simulink model "MECN4029_SIMULINK_BLOCKS_DIAGRAMS"  (R2023b)
settings: Solver=VariableStepAuto  StartTime=0.0  StopTime=815  RelTol=1e-3
PreLoadFcn:
  | Kg=2000;
  | Kt=0.05;
  | Kf=0.05;
  | L=0.006;
  | R=3;
  | J=2.3491;
  | l=1.722;
  | w=1.134;
  | t=0.035;
  | m=21.9;
  | Kd=5;
libraries: slpidlib x2, simulink x1
settings Model: Creator=user  LastModifiedBy=user
settings DataIOCC: ExternalInput=[summertime summerposition]  LoadExternalInput=on

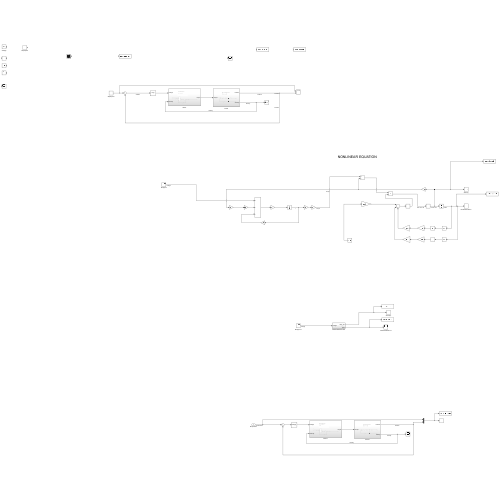
[thumbnail: Simulink's stored preview of the top-level diagram]
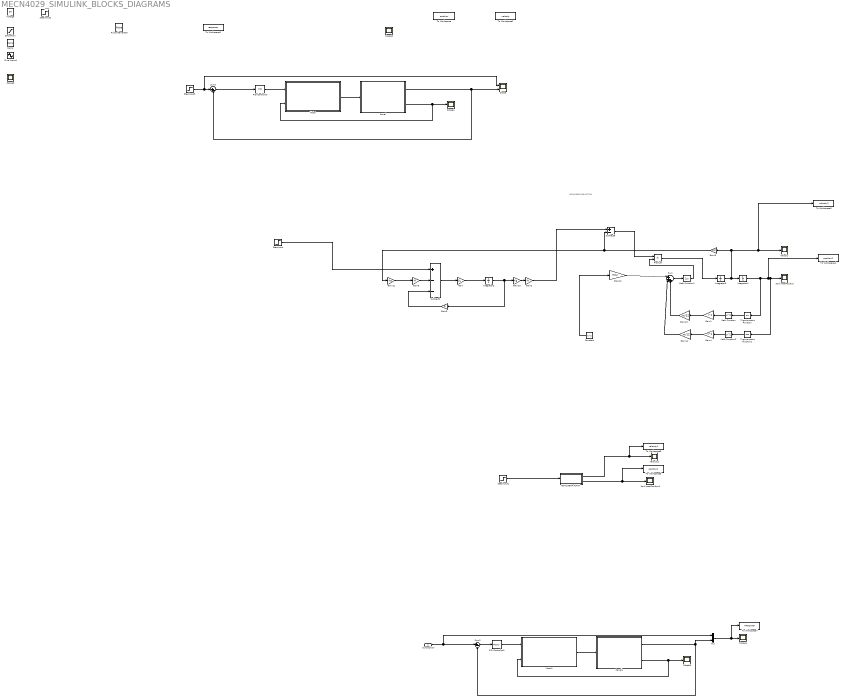
== system MECN4029_SIMULINK_BLOCKS_DIAGRAMS ==
  note: NONLINEAR EQUATION
  Sunposition : Inport
  Constant : Constant  Value=w^2
  Gain : Gain  Gain=1/L
  Gain1 : Gain  Gain=l^2
  Gain10 : Gain  Gain=Kg
  Gain11 : Gain  Gain=Kg
  Gain12 : Gain  Gain=m/12
  Gain13 : Gain  Gain=m/12
  Gain14 : Gain  Gain=m/12
  Gain2 : Gain  Gain=Kt
  Gain3 : Gain  Gain=R
  Gain4 : Gain  Gain=t^2
  Gain5 : Gain  Gain=Kf
  Gain8 : Gain  Gain=Kd
  Integrator1 : Integrator
  Integrator2 : Integrator
  Integrator3 : Integrator
  Math Function : Math  Operator=square
  Math Function1 : Math  Operator=reciprocal
  Math Function2 : Math  Operator=square
  Motor : Subsystem
  Motor1 : Subsystem
  Mux : Mux  Inputs=2
  NON-LINEAR PLANT : Subsystem
  NonlinearPosition : Scope
  NonlinearPosition1 : Scope
  PID Controller : slpidlib/PID Controller  Controller=P  Form=Parallel  TimeDomain=Continuous-time  UseExternalTs=off  SampleTime=-1  IntegratorMethod=Forward Euler  FilterMethod=Forward Euler  ControllerParametersSource=internal  P=200  I=1  UseKiTs=off  D=0  N=100  UseFilter=on  TunerSelectOption=Transfer Function Based (PID Tuner App)  InitialConditionSource=internal  InitialConditionForIntegrator=0  InitialConditionForFilter=0  DifferentiatorICPrevScaledInput=0  ExternalReset=none  TrackingMode=off  Kt=1  LimitOutput=off  SatLimitsSource=internal  UpperSaturationLimit=inf  LowerSaturationLimit=-inf  LinearizeAsGain=on  AntiWindupMode=none  Kb=1  LimitIntegrator=off  UpperIntegratorSaturationLimit=inf  LowerIntegratorSaturationLimit=-inf  POutMin=[]  POutMax=[]  IOutMin=[]  IOutMax=[]  DOutMin=[]  DOutMax=[]  NOutMin=[]  NOutMax=[]  SumOutMin=[]  SumOutMax=[]  SaturationOutMin=[]  SaturationOutMax=[]  PParamMin=[]  PParamMax=[]  IParamMin=[]  IParamMax=[]  DParamMin=[]  DParamMax=[]  NParamMin=[]  NParamMax=[]  KbParamMin=[]  KbParamMax=[]  KtParamMin=[]  KtParamMax=[]  KbOutMin=[]  KbOutMax=[]  KtOutMin=[]  KtOutMax=[]  IntegratorOutMin=[]  IntegratorOutMax=[]  FilterOutMin=[]  FilterOutMax=[]  SumI1OutMin=[]  SumI1OutMax=[]  SumI2OutMin=[]  SumI2OutMax=[]  SumI3OutMin=[]  SumI3OutMax=[]  SumI4OutMin=[]  SumI4OutMax=[]  SumDOutMin=[]  SumDOutMax=[]  DifferentiatorOutMin=[]  DifferentiatorOutMax=[]  FilterDiffOutCoefMin=[]  FilterDiffOutCoefMax=[]  ReciprocalOutMin=[]  ReciprocalOutMax=[]  SumDenOutMin=[]  SumDenOutMax=[]  SumNumOutMin=[]  SumNumOutMax=[]  DivideOutMin=[]  DivideOutMax=[]  UdiffTsProdOutMin=[]  UdiffTsProdOutMax=[]  NTsProdOutMin=[]  NTsProdOutMax=[]  UintegralTsProdOutMin=[]  UintegralTsProdOutMax=[]  UngainTsProdOutMin=[]  UngainTsProdOutMax=[]  ClampingZeroOutDataTypeStr=Inherit: Inherit via back propagation  ClampingZeroOutMin=[]  ClampingZeroOutMax=[]  FilterDenConstantOutDataTypeStr=Inherit: Inherit via back propagation  FilterDenConstantOutMin=[]  FilterDenConstantOutMax=[]  PCopyOutDataTypeStr=Inherit: Inherit via back propagation  PCopyOutMin=[]  PCopyOutMax=[]  NCopyOutDataTypeStr=Inherit: Inherit via back propagation  NCopyOutMin=[]  NCopyOutMax=[]  IntegratorContinuousStateAttributes=''  IntegratorStateMustResolveToSignalObject=off  IntegratorRTWStateStorageClass=Auto  FilterContinuousStateAttributes=''  FilterStateMustResolveToSignalObject=off  FilterRTWStateStorageClass=Auto  ParallelPVariant=InternalParameters  IdealPVariant=Disabled  IVariant=Disabled  DVariant=Disabled  IntegratorVariant=Disabled  SatVariant=Disabled  AWVariant=Disabled  PCopyVariant=Disabled  TRVariant=Disabled  FdbkBlocksVariant=Forward  IdealPFdbkVariant=Disabled  SatFdbkVariant=Disabled  DerivativeFilterVariant=Disabled  NVariant=Disabled  NCopyVariant=Disabled_SignalSpec  FilterICVariant=Disabled  IntegratorICVariant=Disabled  ExternalResetVariant=Disabled  TRSumVariant=Passthrough  SumFdbkVariant=Disabled  SumVariant=Passthrough_P  TsampFilterVariant=InternalTs  TsampNgainVariant=Passthrough  TsampIntegralVariant=Disabled_SignalSpec  ExternalSaturationOutDataTypeStr=Inherit: Same as second input
  PID Controller1 : slpidlib/PID Controller  Controller=PID  Form=Parallel  TimeDomain=Continuous-time  UseExternalTs=off  SampleTime=-1  IntegratorMethod=Forward Euler  FilterMethod=Forward Euler  ControllerParametersSource=internal  P=4922.7881  I=45069.5184  UseKiTs=off  D=-17.6742  N=85.9588  UseFilter=on  TunerSelectOption=Transfer Function Based (PID Tuner App)  InitialConditionSource=internal  InitialConditionForIntegrator=0  InitialConditionForFilter=0  DifferentiatorICPrevScaledInput=0  ExternalReset=none  TrackingMode=off  Kt=1  LimitOutput=off  SatLimitsSource=internal  UpperSaturationLimit=inf  LowerSaturationLimit=-inf  LinearizeAsGain=on  AntiWindupMode=none  Kb=1  LimitIntegrator=off  UpperIntegratorSaturationLimit=inf  LowerIntegratorSaturationLimit=-inf  POutMin=[]  POutMax=[]  IOutMin=[]  IOutMax=[]  DOutMin=[]  DOutMax=[]  NOutMin=[]  NOutMax=[]  SumOutMin=[]  SumOutMax=[]  SaturationOutMin=[]  SaturationOutMax=[]  PParamMin=[]  PParamMax=[]  IParamMin=[]  IParamMax=[]  DParamMin=[]  DParamMax=[]  NParamMin=[]  NParamMax=[]  KbParamMin=[]  KbParamMax=[]  KtParamMin=[]  KtParamMax=[]  KbOutMin=[]  KbOutMax=[]  KtOutMin=[]  KtOutMax=[]  IntegratorOutMin=[]  IntegratorOutMax=[]  FilterOutMin=[]  FilterOutMax=[]  SumI1OutMin=[]  SumI1OutMax=[]  SumI2OutMin=[]  SumI2OutMax=[]  SumI3OutMin=[]  SumI3OutMax=[]  SumI4OutMin=[]  SumI4OutMax=[]  SumDOutMin=[]  SumDOutMax=[]  DifferentiatorOutMin=[]  DifferentiatorOutMax=[]  FilterDiffOutCoefMin=[]  FilterDiffOutCoefMax=[]  ReciprocalOutMin=[]  ReciprocalOutMax=[]  SumDenOutMin=[]  SumDenOutMax=[]  SumNumOutMin=[]  SumNumOutMax=[]  DivideOutMin=[]  DivideOutMax=[]  UdiffTsProdOutMin=[]  UdiffTsProdOutMax=[]  NTsProdOutMin=[]  NTsProdOutMax=[]  UintegralTsProdOutMin=[]  UintegralTsProdOutMax=[]  UngainTsProdOutMin=[]  UngainTsProdOutMax=[]  ClampingZeroOutDataTypeStr=Inherit: Inherit via back propagation  ClampingZeroOutMin=[]  ClampingZeroOutMax=[]  FilterDenConstantOutDataTypeStr=Inherit: Inherit via back propagation  FilterDenConstantOutMin=[]  FilterDenConstantOutMax=[]  PCopyOutDataTypeStr=Inherit: Inherit via back propagation  PCopyOutMin=[]  PCopyOutMax=[]  NCopyOutDataTypeStr=Inherit: Inherit via back propagation  NCopyOutMin=[]  NCopyOutMax=[]  IntegratorContinuousStateAttributes=''  IntegratorStateMustResolveToSignalObject=off  IntegratorRTWStateStorageClass=Auto  FilterContinuousStateAttributes=''  FilterStateMustResolveToSignalObject=off  FilterRTWStateStorageClass=Auto  ParallelPVariant=InternalParameters  IdealPVariant=Disabled  IVariant=InternalParameters  DVariant=InternalParameters  IntegratorVariant=Continuous  SatVariant=Disabled  AWVariant=Passthrough  PCopyVariant=Disabled  TRVariant=Disabled  FdbkBlocksVariant=Forward  IdealPFdbkVariant=Disabled  SatFdbkVariant=Disabled  DerivativeFilterVariant=ContFilter  NVariant=InternalParameters  NCopyVariant=Disabled  FilterICVariant=InternalICsFilter  IntegratorICVariant=InternalICs  ExternalResetVariant=Disabled  TRSumVariant=Passthrough  SumFdbkVariant=Disabled  SumVariant=Sum_PID  TsampFilterVariant=InternalTs  TsampNgainVariant=Passthrough  TsampIntegralVariant=Disabled_SignalSpec  ExternalSaturationOutDataTypeStr=Inherit: Same as second input
  Panel : Subsystem
  Panel1 : Subsystem
  Product : Product
  Pulse Generator : DiscretePulseGenerator  PulseType=Time based  Amplitude=30  Period=0.05  PulseWidth=5  PhaseDelay=0.01  VectorParams1D=off
  Ramp : simulink/Sources/Ramp  slope=5  start=1  InitialOutput=0
  Saturation : Saturate  UpperLimit=30  LowerLimit=-30
  Scope : Scope  NumInputPorts=2
  Scope{1..5} (5 alike) : Scope
  Sine Wave1 : Sin  Amplitude=30  SampleTime=0
  StepInput : Step  Time=0.01  After=30  SampleTime=0
  StepInput1 : Step  Time=0.01  After=30  SampleTime=0
  StepInput2 : Step  Time=0.01  After=30  SampleTime=0
  StepInput3 : Step  After=30  SampleTime=0
  Subtract1 : Sum  Inputs=+--
  Subtract3 : Sum  Inputs=+-
  Sum : Sum  Inputs=|+++  OutDataTypeStr=Inherit: Keep MSB
  Sum1 : Sum  Inputs=|+-
  Sum2 : Sum  Inputs=|+-
  To Workspace : ToWorkspace  VariableName=position  SampleTime=-1
  To Workspace1 : ToWorkspace  VariableName=velocity  SampleTime=-1
  To Workspace2 : ToWorkspace  VariableName=response  SampleTime=-1
  To Workspace3 : ToWorkspace  VariableName=velocity2  SampleTime=-1
  To Workspace4 : ToWorkspace  VariableName=position2  SampleTime=-1
  To Workspace5 : ToWorkspace  VariableName=velocity1  SampleTime=-1
  To Workspace6 : ToWorkspace  VariableName=position1  SampleTime=-1
  To Workspace7 : ToWorkspace  VariableName=TRACKING  SampleTime=-1
  Trigonometric Function : Trigonometry
  Trigonometric Function1 : Trigonometry  Operator=cos
  Velocity : Scope
  Velocity1 : Scope
  Voltage : Constant  Value=30
  wires:
  Panel/1(Position) -> Sum1/2, Scope/2  "Position"
  Panel/2(Velocity) -> Scope1/1, Motor/2(Velocity)  "Velocity"
  Motor/1(torque) -> Panel/1(Torque)
  Integrator1/1 -> Trigonometric Function/1, To Workspace4/1, Trigonometric Function1/1, NonlinearPosition/1  "theta"
  Integrator3/1 -> Gain8/1, To Workspace3/1, Velocity/1, Integrator1/1  "theta_dot"
  Gain8/1 -> Gain11/1, Subtract3/2
  Gain/1 -> Integrator2/1
  Integrator2/1 -> Gain10/1, Gain3/1  "i"
  Gain3/1 -> Subtract1/3
  Gain5/1 -> Subtract1/2
  Subtract1/1 -> Gain/1
  Gain2/1 -> Subtract3/1  "torque"
  Constant/1 -> Gain12/1
  Math Function2/1 -> Gain4/1
  Math Function/1 -> Gain1/1
  Trigonometric Function/1 -> Math Function/1
  Math Function1/1 -> Product/2
  Sum/1 -> Math Function1/1
  Trigonometric Function1/1 -> Math Function2/1
  Product/1 -> Integrator3/1  "theta_dot_dot"
  Subtract3/1 -> Product/1
  Gain10/1 -> Gain2/1
  Gain11/1 -> Gain5/1
  Gain12/1 -> Sum/1
  Gain13/1 -> Sum/3
  Gain14/1 -> Sum/2
  Gain1/1 -> Gain13/1
  Gain4/1 -> Gain14/1
  Sum1/1 -> PID Controller/1  "Voltage"
  NON-LINEAR PLANT/2(theta) -> NonlinearPosition1/1, To Workspace6/1
  NON-LINEAR PLANT/1(theta_dot) -> To Workspace5/1, Velocity1/1
  StepInput1/1 -> NON-LINEAR PLANT/1(Voltage)  "Voltage"
  StepInput/1 -> Subtract1/1  "Voltage"
  StepInput3/1 -> Scope/1, Sum1/1
  PID Controller/1 -> Motor/1(Voltage)
  Sunposition/1 -> Sum2/1, Mux/1  "SunPosition"
  Motor1/1(torque) -> Panel1/1(Torque)
  Panel1/1(Position) -> Mux/2, Sum2/2  "Position"
  Panel1/2(Velocity) -> Scope5/1, Motor1/2(Velocity)  "Velocity"
  Mux/1 -> To Workspace7/1, Scope4/1
  Sum2/1 -> PID Controller1/1
  PID Controller1/1 -> Motor1/1(Voltage)

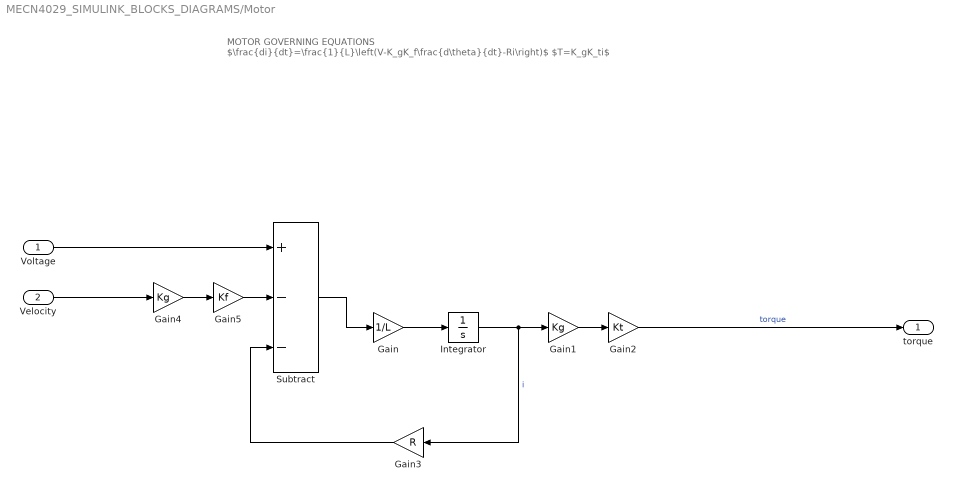
== system MECN4029_SIMULINK_BLOCKS_DIAGRAMS/Motor ==
  note: MOTOR GOVERNING EQUATIONS $\frac{di}{dt}=\frac{1}{L}\left(V-K_gK_f\frac{d\theta}{dt}-Ri\right)$
      | $T=K_gK_ti$
  Voltage : Inport
  Velocity : Inport  Port=2
  Gain : Gain  Gain=1/L
  Gain1 : Gain  Gain=Kg
  Gain2 : Gain  Gain=Kt
  Gain3 : Gain  Gain=R
  Gain4 : Gain  Gain=Kg
  Gain5 : Gain  Gain=Kf
  Integrator : Integrator
  Subtract : Sum  Inputs=+--
  torque : Outport
  wires:
  Gain3/1 -> Subtract/3
  Gain5/1 -> Subtract/2
  Gain/1 -> Integrator/1
  Integrator/1 -> Gain1/1, Gain3/1  "i"
  Subtract/1 -> Gain/1
  Velocity/1 -> Gain4/1
  Gain2/1 -> torque/1  "torque"
  Voltage/1 -> Subtract/1
  Gain1/1 -> Gain2/1
  Gain4/1 -> Gain5/1

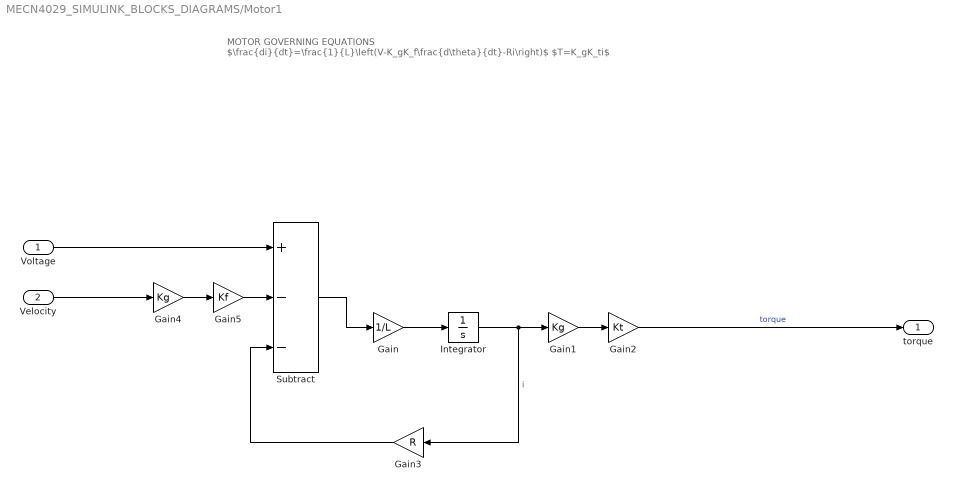
== system MECN4029_SIMULINK_BLOCKS_DIAGRAMS/Motor1 ==
  note: MOTOR GOVERNING EQUATIONS $\frac{di}{dt}=\frac{1}{L}\left(V-K_gK_f\frac{d\theta}{dt}-Ri\right)$
      | $T=K_gK_ti$
  Voltage : Inport
  Velocity : Inport  Port=2
  Gain : Gain  Gain=1/L
  Gain1 : Gain  Gain=Kg
  Gain2 : Gain  Gain=Kt
  Gain3 : Gain  Gain=R
  Gain4 : Gain  Gain=Kg
  Gain5 : Gain  Gain=Kf
  Integrator : Integrator
  Subtract : Sum  Inputs=+--
  torque : Outport
  wires:
  Gain3/1 -> Subtract/3
  Gain5/1 -> Subtract/2
  Gain/1 -> Integrator/1
  Integrator/1 -> Gain1/1, Gain3/1  "i"
  Subtract/1 -> Gain/1
  Velocity/1 -> Gain4/1
  Gain2/1 -> torque/1  "torque"
  Voltage/1 -> Subtract/1
  Gain1/1 -> Gain2/1
  Gain4/1 -> Gain5/1

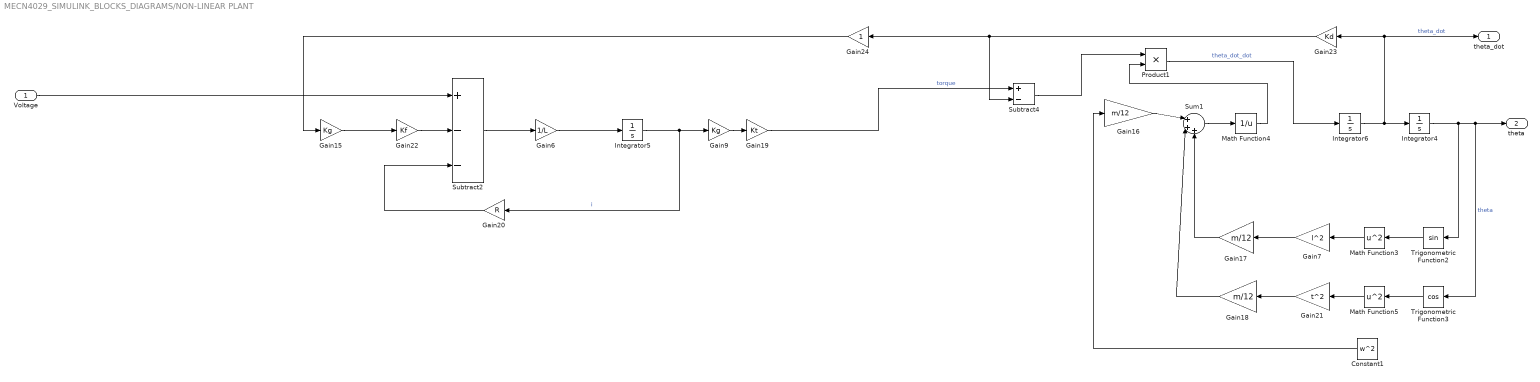
== system MECN4029_SIMULINK_BLOCKS_DIAGRAMS/NON-LINEAR PLANT ==
  Voltage : Inport
  Constant1 : Constant  Value=w^2
  Gain15 : Gain  Gain=Kg
  Gain16 : Gain  Gain=m/12
  Gain17 : Gain  Gain=m/12
  Gain18 : Gain  Gain=m/12
  Gain19 : Gain  Gain=Kt
  Gain20 : Gain  Gain=R
  Gain21 : Gain  Gain=t^2
  Gain22 : Gain  Gain=Kf
  Gain23 : Gain  Gain=Kd
  Gain24 : Gain
  Gain6 : Gain  Gain=1/L
  Gain7 : Gain  Gain=l^2
  Gain9 : Gain  Gain=Kg
  Integrator4 : Integrator
  Integrator5 : Integrator
  Integrator6 : Integrator
  Math Function3 : Math  Operator=square
  Math Function4 : Math  Operator=reciprocal
  Math Function5 : Math  Operator=square
  Product1 : Product
  Subtract2 : Sum  Inputs=+--
  Subtract4 : Sum  Inputs=+-
  Sum1 : Sum  Inputs=|+++  OutDataTypeStr=Inherit: Keep MSB
  Trigonometric Function2 : Trigonometry
  Trigonometric Function3 : Trigonometry  Operator=cos
  theta_dot : Outport
  theta : Outport  Port=2
  wires:
  Trigonometric Function3/1 -> Math Function5/1
  Gain7/1 -> Gain17/1
  Gain6/1 -> Integrator5/1
  Gain15/1 -> Gain22/1
  Constant1/1 -> Gain16/1
  Gain24/1 -> Gain15/1
  Subtract4/1 -> Product1/1
  Gain21/1 -> Gain18/1
  Math Function4/1 -> Product1/2
  Gain22/1 -> Subtract2/2
  Gain18/1 -> Sum1/2
  Integrator6/1 -> theta_dot/1, Gain23/1, Integrator4/1  "theta_dot"
  Math Function3/1 -> Gain7/1
  Integrator4/1 -> theta/1, Trigonometric Function3/1, Trigonometric Function2/1  "theta"
  Integrator5/1 -> Gain9/1, Gain20/1  "i"
  Product1/1 -> Integrator6/1  "theta_dot_dot"
  Gain16/1 -> Sum1/1
  Gain20/1 -> Subtract2/3
  Gain9/1 -> Gain19/1
  Subtract2/1 -> Gain6/1
  Gain17/1 -> Sum1/3
  Gain23/1 -> Gain24/1, Subtract4/2
  Sum1/1 -> Math Function4/1
  Voltage/1 -> Subtract2/1
  Trigonometric Function2/1 -> Math Function3/1
  Gain19/1 -> Subtract4/1  "torque"
  Math Function5/1 -> Gain21/1

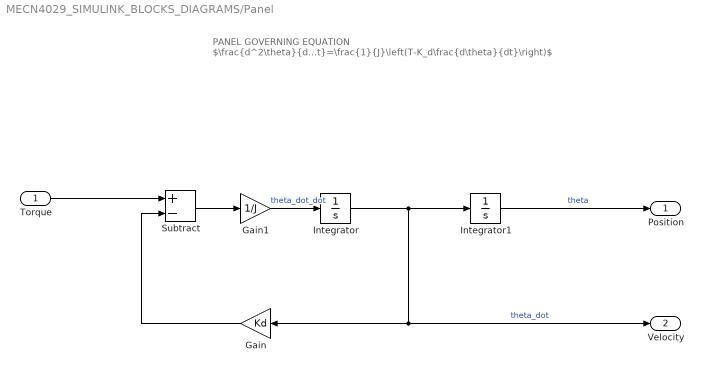
== system MECN4029_SIMULINK_BLOCKS_DIAGRAMS/Panel ==
  note: PANEL GOVERNING EQUATION
      | $\frac{d^2\theta}{dt}=\frac{1}{J}\left(T-K_d\frac{d\theta}{dt}\right)$
  Torque : Inport
  Gain : Gain  Gain=Kd
  Gain1 : Gain  Gain=1/J
  Integrator : Integrator
  Integrator1 : Integrator
  Subtract : Sum  Inputs=+-
  Position : Outport
  Velocity : Outport  Port=2
  wires:
  Integrator1/1 -> Position/1  "theta"
  Integrator/1 -> Velocity/1, Gain/1, Integrator1/1  "theta_dot"
  Gain/1 -> Subtract/2
  Torque/1 -> Subtract/1
  Subtract/1 -> Gain1/1
  Gain1/1 -> Integrator/1  "theta_dot_dot"

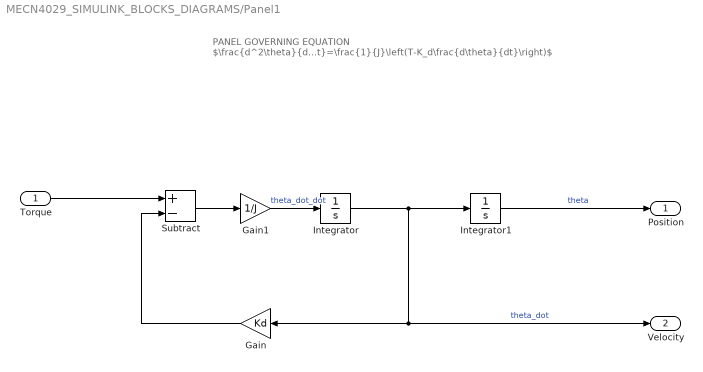
== system MECN4029_SIMULINK_BLOCKS_DIAGRAMS/Panel1 ==
  note: PANEL GOVERNING EQUATION
      | $\frac{d^2\theta}{dt}=\frac{1}{J}\left(T-K_d\frac{d\theta}{dt}\right)$
  Torque : Inport
  Gain : Gain  Gain=Kd
  Gain1 : Gain  Gain=1/J
  Integrator : Integrator
  Integrator1 : Integrator
  Subtract : Sum  Inputs=+-
  Position : Outport
  Velocity : Outport  Port=2
  wires:
  Integrator1/1 -> Position/1  "theta"
  Integrator/1 -> Velocity/1, Gain/1, Integrator1/1  "theta_dot"
  Gain/1 -> Subtract/2
  Torque/1 -> Subtract/1
  Subtract/1 -> Gain1/1
  Gain1/1 -> Integrator/1  "theta_dot_dot"
